simulink model "o_heli3d"  (Simulink 7.7)
settings: Solver=ode1  StartTime=0.0  StopTime=inf  FixedStep=0.002  RelTol=1e-3
values from neighbouring files (symbols this model uses):
  A_kal = Kest.a    [setup_lab_heli_3d_various_controler_with_Kalman_Filter.m]
  B_kal = Kest.b    [setup_lab_heli_3d_various_controler_with_Kalman_Filter.m]
  C = [1,0,0,0,0,0 ... (first row only)    [lab_init.m]    (also in o_lqi.m = [1,0,0,0,0; 0,0,0,0,1])
  C_kal = eye(6)    [setup_lab_heli_3d_various_controler_with_Kalman_Filter.m]
  CMD_ELEV_POS_LIMIT_LOWER = elev_0*180/pi    (= -27.5)    [setup_lab_heli_3d.m]    (also in setup_lab_heli_3d_simple.m; setup_lab_heli_3d_various_controler.m; setup_lab_heli_3d_various_controler_with_Kalman_Filter.m)
  CMD_ELEV_POS_LIMIT_UPPER = -CMD_ELEV_POS_LIMIT_LOWER    (= 27.5)    [setup_lab_heli_3d.m]    (also in setup_lab_heli_3d_simple.m; setup_lab_heli_3d_various_controler.m; setup_lab_heli_3d_various_controler_with_Kalman_Filter.m)
  CMD_RATE_LIMIT = 45.0 * pi / 180    (= 0.785398163397)    [setup_lab_heli_3d.m]    (also in setup_lab_heli_3d_simple.m; setup_lab_heli_3d_various_controler.m; setup_lab_heli_3d_various_controler_with_Kalman_Filter.m)
  D_kal = zeros(6,5)    [setup_lab_heli_3d_various_controler_with_Kalman_Filter.m]
  elev_0 = -27.5*pi/180    (= -0.479965544298)    [setup_lab_heli_3d.m]    (also in setup_lab_heli_3d_simple.m; setup_lab_heli_3d_various_controler.m; setup_lab_heli_3d_various_controler_with_Kalman_Filter.m)
  g = 9.81    [linnlsys.m]
  K_AMP = 3    [setup_lab_heli_3d.m]    (also in setup_lab_heli_3d_simple.m; setup_lab_heli_3d_various_controler.m; setup_lab_heli_3d_various_controler_with_Kalman_Filter.m)
  K_JOYSTICK_X = 40.0    (= 40)    [setup_lab_heli_3d.m]    (also in setup_lab_heli_3d_simple.m; setup_lab_heli_3d_various_controler.m; setup_lab_heli_3d_various_controler_with_Kalman_Filter.m)
  K_JOYSTICK_Y = 45.0    (= 45)    [setup_lab_heli_3d.m]    (also in setup_lab_heli_3d_simple.m; setup_lab_heli_3d_various_controler.m; setup_lab_heli_3d_various_controler_with_Kalman_Filter.m)
  Kr = [L(:,1),L(:,5)]    [o_lqi.m]    (also in setup_lab_heli_3d_various_controler.m = [L eye(2,2)]*A_tot_inv*[zeros(6,3);eye(3,3)]; setup_lab_heli_3d_various_controler_with_Kalman_Filter.m = -V_svd*inv(S_svd)*U_svd')
  L = lqr( Ae, Be, Q, R )    [o_lqi.m]    (also in setup_lab_heli_3d_various_controler.m = Le(:,1:6); setup_lab_heli_3d_various_controler_with_Kalman_Filter.m = lqr( A, B, Q, R ))
  La = 26.0 * 0.0254    (= 0.6604)    [linnlsys.m]
  V = eye(3)    [setup_lab_heli_3d_various_controler_with_Kalman_Filter.m]
  VMAX_AMP = 24    [setup_lab_heli_3d.m]    (also in setup_lab_heli_3d_simple.m; setup_lab_heli_3d_various_controler.m; setup_lab_heli_3d_various_controler_with_Kalman_Filter.m)
  VMAX_DAC = 10    [setup_lab_heli_3d.m]    (also in setup_lab_heli_3d_simple.m; setup_lab_heli_3d_various_controler.m; setup_lab_heli_3d_various_controler_with_Kalman_Filter.m)
  W = diag([1e3 1e3 1e3 1e-3 1e-3 1e-3])    [setup_lab_heli_3d_various_controler_with_Kalman_Filter.m]
  wcf = 2 * pi * 2.5    (= 15.7079632679)    [setup_ads_configuration.m]    (also in setup_lab_heli_3d.m = 125.663706144; setup_lab_heli_3d_simple.m = 125.663706144; setup_lab_heli_3d_various_controler.m = 125.663706144; setup_lab_heli_3d_various_controler_with_Kalman_Filter.m = 125.663706144)
  zetaf = 0.9    [setup_lab_heli_3d.m]    (also in setup_lab_heli_3d_simple.m; setup_lab_heli_3d_various_controler.m; setup_lab_heli_3d_various_controler_with_Kalman_Filter.m)
undefined symbols (not defined in the file or in its folder): ax, ay, az, CMD_TRAVEL_POS_LIMIT_LOWER, CMD_TRAVEL_POS_LIMIT_UPPER, HIL, K_EC_E, K_EC_P, K_EC_T, Kf, Lw, m_b, m_f, m_w, P, p, qc_get_step_size
libraries: quarc_library x5, simulink_extras x4, simulink x3
settings Model: Creator=MLevis  LastModifiedBy=helicopter  SimulationMode=external  ExtModeTrigDuration=10000
settings SolverCC: PositivePriorityOrder=on
settings OptimizationCC: InitFltsAndDblsToZero=on
settings DebuggingCC: SaveWithParameterizedLinksMsg=none  StrictBusMsg=Warning
settings RTWCC: SystemTargetFile=quarc_win64.tlc  TemplateMakefile=quarc_default_tmf  Description=QUARC Win64 Target  ProcessScript=quarc_win64_make_rtw_hook
settings STFCustomTargetCC: TargetPreCompLibLocation=C:\PROGRA~3\QUARC\lib\2011a\win64\release  FunctionExecutionProfile=off  GeneratePreprocessorConditionals=Disable all  SystemTargetFile=quarc_win64.tlc
settings GRTTargetCC: TargetPreCompLibLocation=C:\PROGRA~3\QUARC\lib\2011a\win64\release  ParMdlRefBuildCompliant=off  CompOptLevelCompliant=off  MatFileLogging=off  ExtMode=on  ExtModeMexFile=quarc_comm

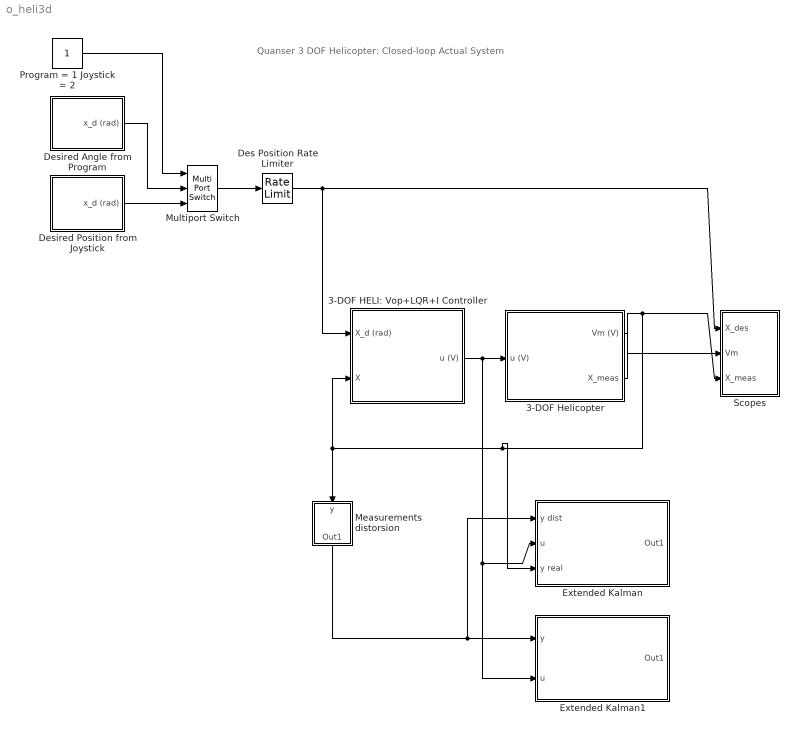
== system o_heli3d ==
  note: Quanser 3 DOF Helicopter:
      | Closed-loop Actual System
  3-DOF HELI: Vop+LQR+I Controller : Subsystem
  3-DOF Helicopter : Subsystem
  Des Position Rate Limiter : RateLimiter  RisingSlewLimit=CMD_RATE_LIMIT  FallingSlewLimit=-CMD_RATE_LIMIT  SampleTimeMode=inherited
  Desired Angle from Program : Subsystem
  Desired Position from Joystick : Subsystem
  Extended Kalman : Subsystem
  Extended Kalman1 : Subsystem
  Measurements distorsion : Subsystem
  Multiport Switch : MultiPortSwitch  Inputs=2  zeroidx=off
  Program = 1 Joystick = 2 : Constant
  Scopes : Subsystem
  wires:
  3-DOF Helicopter/1(Vm (V)) -> Scopes/2(Vm)
  3-DOF Helicopter/2(X_meas) -> Scopes/3(X_meas), 3-DOF HELI: Vop+LQR+I Controller/2(X), Measurements distorsion/1(y), Extended Kalman/3(y real)
  Des Position Rate Limiter/1 -> Scopes/1(X_des), 3-DOF HELI: Vop+LQR+I Controller/1(X_d (rad))
  Program = 1 Joystick = 2/1 -> Multiport Switch/1
  Desired Angle from Program/1(x_d (rad)) -> Multiport Switch/2
  Desired Position from Joystick/1(x_d (rad)) -> Multiport Switch/3
  Multiport Switch/1 -> Des Position Rate Limiter/1
  3-DOF HELI: Vop+LQR+I Controller/1(u (V)) -> 3-DOF Helicopter/1(u (V)), Extended Kalman1/2(u), Extended Kalman/2(u)
  Measurements distorsion/1(Out1) -> Extended Kalman1/1(y), Extended Kalman/1(y dist)

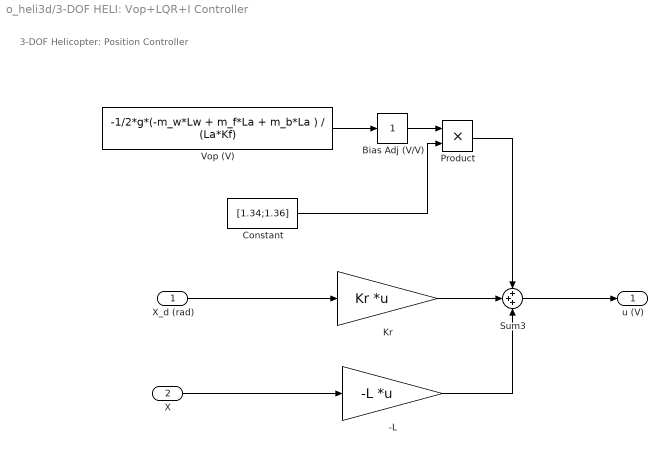
== system o_heli3d/3-DOF HELI: Vop+LQR+I Controller ==
  note: 3-DOF Helicopter: Position Controller
  X_d (rad) : Inport
  X : Inport  Port=2
  -L : Gain  Gain=-L  Multiplication=Matrix(K*u)
  Bias Adj (V/V) : simulink/Math Operations/Slider Gain  SystemSampleTime=-1  low=0  gain=1  high=1
  Constant : Constant  Value=[1.34;1.36]
  Kr : Gain  Gain=Kr  Multiplication=Matrix(K*u)
  Product : Product  RndMeth=Zero
  Sum3 : Sum  Inputs=+++
  Vop (V) : Constant  Value=-1/2*g*(-m_w*Lw + m_f*La + m_b*La ) / (La*Kf)
  u (V) : Outport
  wires:
  X_d (rad)/1 -> Kr/1
  X/1 -> -L/1
  Sum3/1 -> u (V)/1
  Vop (V)/1 -> Bias Adj (V/V)/1
  Bias Adj (V/V)/1 -> Product/1
  Constant/1 -> Product/2
  Product/1 -> Sum3/1
  Kr/1 -> Sum3/2
  -L/1 -> Sum3/3

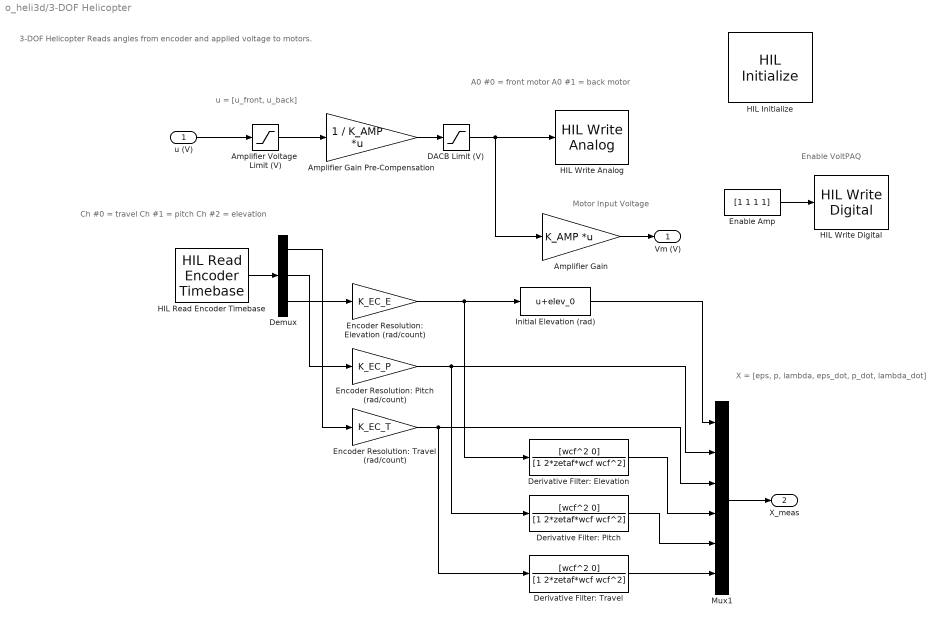
== system o_heli3d/3-DOF Helicopter ==
  note: A0 #0 = front motor
      | A0 #1 = back motor
  note: u = [u_front, u_back]
  note: Motor Input Voltage
  note: 3-DOF Helicopter
      | Reads angles from encoder and applied voltage to motors.
  note: Ch #0 = travel
      | Ch #1 = pitch
      | Ch #2 = elevation
  note: X = [eps, p, lambda, eps_dot, p_dot, lambda_dot]
  note: Enable VoltPAQ
  u (V) : Inport
  Amplifier Gain : Gain  Gain=K_AMP  Multiplication=Matrix(K*u)  SaturateOnIntegerOverflow=on  OutDataTypeStr=Inherit: Same as input  ParamDataTypeStr=Inherit: Same as input
  Amplifier Gain Pre-Compensation : Gain  Gain=1 / K_AMP  Multiplication=Matrix(K*u)  SaturateOnIntegerOverflow=on  OutDataTypeStr=Inherit: Same as input  ParamDataTypeStr=Inherit: Same as input
  Amplifier Voltage  Limit (V) : Saturate  UpperLimit=VMAX_AMP  LowerLimit=-VMAX_AMP
  DACB Limit (V) : Saturate  UpperLimit=VMAX_DAC  LowerLimit=-VMAX_DAC
  Demux : Demux  Outputs=3
  Derivative Filter: Elevation : TransferFcn  Numerator=[wcf^2 0]  Denominator=[1 2*zetaf*wcf wcf^2]
  Derivative Filter: Pitch : TransferFcn  Numerator=[wcf^2 0]  Denominator=[1 2*zetaf*wcf wcf^2]
  Derivative Filter: Travel : TransferFcn  Numerator=[wcf^2 0]  Denominator=[1 2*zetaf*wcf wcf^2]
  Enable Amp : Constant  Value=[1 1 1 1]
  Encoder Resolution: Elevation (rad/count) : Gain  Gain=K_EC_E
  Encoder Resolution: Pitch (rad/count) : Gain  Gain=K_EC_P
  Encoder Resolution: Travel (rad/count) : Gain  Gain=K_EC_T
  HIL Initialize : quarc_library/Data Acquisition/Generic/Configuration/HIL Initialize  object_name=HIL-1  board_type=q8_usb  board_number=0  board_options=update_rate=normal  exclusive=off  active=on  hardware_clocks=[0:2]  clock_modes=[]  initial_clock_frequencies=[]  set_clock_params_at_start=off  set_clock_params_at_switch_in=off  set_clock_frequencies_at_start=off  set_clock_frequencies_at_switch_in=off  analog_input_channels=[0:7]  analog_input_maximums=10  analog_input_minimums=-10  set_analog_input_params_at_start=on  set_analog_input_params_at_switch_in=off  analog_output_channels=[0:7]  analog_output_maximums=10  analog_output_minimums=-10  initial_analog_outputs=[0]  final_analog_outputs=[0]  watchdog_analog_outputs=0  set_analog_output_params_at_start=on  set_analog_output_params_at_switch_in=off  set_analog_outputs_at_start=on  set_analog_outputs_at_switch_in=off  set_analog_outputs_at_terminate=on  set_analog_outputs_at_switch_out=off  set_analog_outputs_on_watchdog=off  digital_input_channels=[4:7]  digital_output_channels=[0:3]  digital_output_configuration=[]  initial_digital_outputs=[0]  final_digital_outputs=[0]  watchdog_digital_outputs=[0]  set_digital_output_params_at_start=off  set_digital_output_params_at_switch_in=off  set_digital_outputs_at_start=on  set_digital_outputs_at_switch_in=off  set_digital_outputs_at_terminate=on  set_digital_outputs_at_switch_out=off  set_digital_outputs_on_watchdog=off  encoder_channels=[0:7]  quadrature=[4]  encoder_filter_frequency=[]  initial_encoder_counts=[0]  set_encoder_params_at_start=on  set_encoder_params_at_switch_in=off  set_encoder_counts_at_start=on  set_encoder_counts_at_switch_in=off  pwm_channels=[0:7]  pwm_modes=0  pwm_frequency=99.532799999999995e6/4095  pwm_configuration=[0]  pwm_alignment=[0]  pwm_polarity=[1]  pwm_leading_deadband=[0]  pwm_trailing_deadband=[0]  initial_pwm_outputs=[0]  final_pwm_outputs=[0]  watchdog_pwm_outputs=[0]  set_pwm_params_at_start=on  set_pwm_params_at_switch_in=off  set_pwm_outputs_at_start=on  set_pwm_outputs_at_switch_in=off  set_pwm_outputs_at_terminate=on  set_pwm_outputs_at_switch_out=off  set_pwm_outputs_on_watchdog=off  other_output_channels=[]  initial_other_outputs=[]  final_other_outputs=[]  watchdog_other_outputs=[]  set_other_outputs_at_start=off  set_other_outputs_at_switch_in=off  set_other_outputs_at_terminate=off  set_other_outputs_at_switch_out=off  set_other_outputs_on_watchdog=off
  HIL Read Encoder Timebase : quarc_library/Data Acquisition/Generic/Timebases/HIL Read Encoder Timebase  object_name=HIL-1  clock=0  channels=[0:2]  samples_in_buffer=max(ceil(1/qc_get_step_size), 1)  active=on  vector_output=on  data_type_mode=Inherit via back propagation  data_type=double
  HIL Write Analog : quarc_library/Data Acquisition/Generic/Immediate I//O/HIL Write Analog  object_name=HIL-1  channels=[0,1]  sample_time=-1  active=off  vector_input=on
  HIL Write Digital : quarc_library/Data Acquisition/Generic/Immediate I//O/HIL Write Digital  object_name=HIL-1  channels=[0:3]  sample_time=-1  active=off  vector_input=on
  Initial Elevation (rad) : Bias  Bias=elev_0
  Mux1 : Mux  Inputs=6
  Vm (V) : Outport
  X_meas : Outport  Port=2
  wires:
  HIL Read Encoder Timebase/1 -> Demux/1
  Mux1/1 -> X_meas/1
  Amplifier Gain Pre-Compensation/1 -> DACB Limit (V)/1
  Amplifier Voltage  Limit (V)/1 -> Amplifier Gain Pre-Compensation/1
  Amplifier Gain/1 -> Vm (V)/1
  u (V)/1 -> Amplifier Voltage  Limit (V)/1
  DACB Limit (V)/1 -> Amplifier Gain/1, HIL Write Analog/1
  Demux/3 -> Encoder Resolution: Elevation (rad/count)/1
  Demux/1 -> Encoder Resolution: Travel (rad/count)/1
  Demux/2 -> Encoder Resolution: Pitch (rad/count)/1
  Encoder Resolution: Elevation (rad/count)/1 -> Derivative Filter: Elevation/1, Initial Elevation (rad)/1
  Encoder Resolution: Pitch (rad/count)/1 -> Mux1/2, Derivative Filter: Pitch/1
  Encoder Resolution: Travel (rad/count)/1 -> Mux1/3, Derivative Filter: Travel/1
  Derivative Filter: Elevation/1 -> Mux1/4
  Derivative Filter: Pitch/1 -> Mux1/5
  Derivative Filter: Travel/1 -> Mux1/6
  Initial Elevation (rad)/1 -> Mux1/1
  Enable Amp/1 -> HIL Write Digital/1

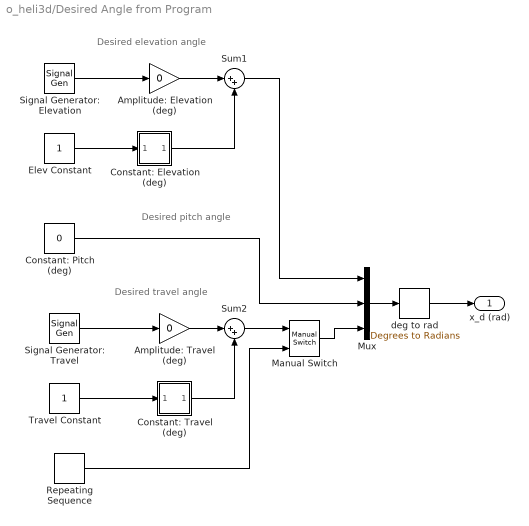
== system o_heli3d/Desired Angle from Program ==
  note: Desired travel angle
  note: Desired elevation angle
  note: Desired pitch angle
  Amplitude: Elevation (deg) : Gain  Gain=0
  Amplitude: Travel (deg) : Gain  Gain=0
  Constant: Elevation (deg) : Subsystem  LoadFcn=slideg Load  StartFcn=slideg StartFcn  StopFcn=slideg StopFcn  mask(Slider Gain){low=-27.5, gain=0, high=100}
      settings: CopyFcn=slideg Copy  DeleteFcn=slideg DeleteBlock  NameChangeFcn=slideg NameChange  OpenFcn=slideg Open  CloseFcn=slideg Close  ParentCloseFcn=slideg ParentClose
      mask Display: disp(gain)
  Constant: Pitch (deg) : Constant  Value=0
  Constant: Travel (deg) : Subsystem  LoadFcn=slideg Load  StartFcn=slideg StartFcn  StopFcn=slideg StopFcn  mask(Slider Gain){low=-90, gain=0, high=90}
      settings: CopyFcn=slideg Copy  DeleteFcn=slideg DeleteBlock  NameChangeFcn=slideg NameChange  OpenFcn=slideg Open  CloseFcn=slideg Close  ParentCloseFcn=slideg ParentClose
      mask Display: disp(gain)
  Elev Constant : Constant
  Manual Switch : simulink/Signal Routing/Manual Switch  SystemSampleTime=-1  sw=1  action=0  varsize=off
  Mux : Mux  Inputs=3
  Repeating Sequence : simulink/Sources/Repeating Sequence  SystemSampleTime=-1  rep_seq_t="[0  15 16  30  45  46 60 ]"  rep_seq_y="[0 0 30 30  30 0 0 ]"
  Signal Generator: Elevation : SignalGenerator  WaveForm=square  Frequency=0.04
  Signal Generator: Travel : SignalGenerator  WaveForm=square  Frequency=0.03
  Sum1 : Sum  Inputs=|++
  Sum2 : Sum  Inputs=|++
  Travel Constant : Constant
  deg to rad : simulink_extras/Transformations/Degrees to Radians  SystemSampleTime=-1
  x_d (rad) : Outport
  wires:
  deg to rad/1 -> x_d (rad)/1
  Signal Generator: Travel/1 -> Amplitude: Travel (deg)/1
  Amplitude: Travel (deg)/1 -> Sum2/1
  Travel Constant/1 -> Constant: Travel (deg)/1(In1)
  Sum1/1 -> Mux/1
  Signal Generator: Elevation/1 -> Amplitude: Elevation (deg)/1
  Amplitude: Elevation (deg)/1 -> Sum1/1
  Mux/1 -> deg to rad/1
  Constant: Pitch (deg)/1 -> Mux/2
  Elev Constant/1 -> Constant: Elevation (deg)/1(In1)
  Constant: Elevation (deg)/1(Out1) -> Sum1/2
  Constant: Travel (deg)/1(Out1) -> Sum2/2
  Sum2/1 -> Manual Switch/1
  Manual Switch/1 -> Mux/3
  Repeating Sequence/1 -> Manual Switch/2

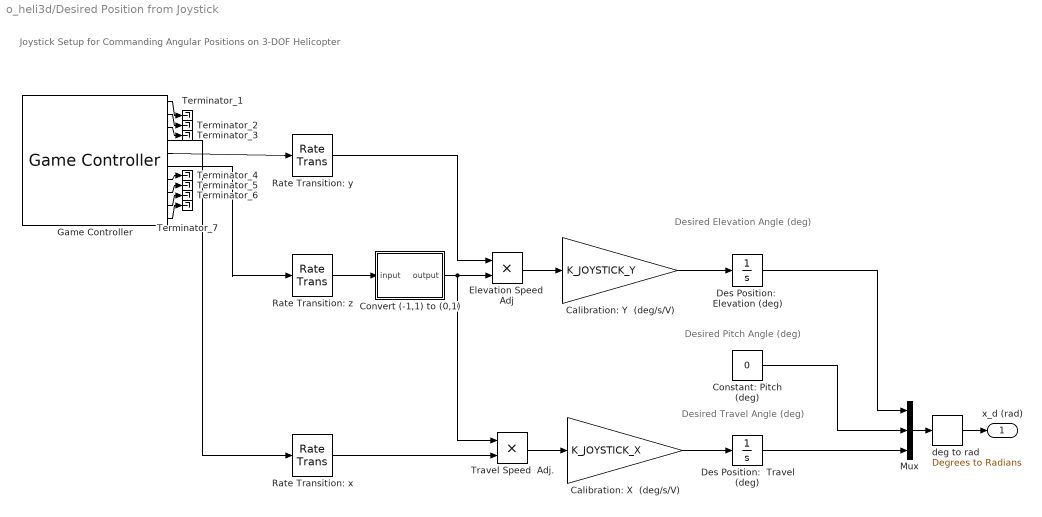
== system o_heli3d/Desired Position from Joystick ==
  note: Desired Pitch Angle (deg)
  note: Desired Elevation Angle (deg)
  note: Desired Travel Angle (deg)
  note: Joystick Setup for Commanding Angular Positions on 3-DOF Helicopter
  Calibration: X  (deg/s/V) : Gain  Gain=K_JOYSTICK_X
  Calibration: Y  (deg/s/V) : Gain  Gain=K_JOYSTICK_Y
  Constant: Pitch (deg) : Constant  Value=0
  Convert (-1,1) to (0,1) : Subsystem
  Des Position:  Elevation (deg) : Integrator  InitialCondition=elev_0*180/pi  LimitOutput=on  UpperSaturationLimit=CMD_ELEV_POS_LIMIT_UPPER  LowerSaturationLimit=CMD_ELEV_POS_LIMIT_LOWER
  Des Position:  Travel (deg) : Integrator  UpperSaturationLimit=CMD_TRAVEL_POS_LIMIT_UPPER  LowerSaturationLimit=CMD_TRAVEL_POS_LIMIT_LOWER
  Elevation Speed  Adj : Product  RndMeth=Zero
  Game Controller : quarc_library/Devices/Peripherals/Target/Game Controller  controller=1  buffer_size=12  deadzone=[]  saturation=[]  sample_time=max(qc_get_step_size, 0.01)  auto_center=off  enabled=on
  Mux : Mux  Inputs=3
  Rate Transition: x : RateTransition
  Rate Transition: y : RateTransition
  Rate Transition: z : RateTransition
  Terminator_{1..7} (7 alike) : Terminator
  Travel Speed  Adj. : Product  RndMeth=Zero
  deg to rad : simulink_extras/Transformations/Degrees to Radians  SystemSampleTime=-1
  x_d (rad) : Outport
  wires:
  Des Position:  Elevation (deg)/1 -> Mux/1
  Constant: Pitch (deg)/1 -> Mux/2
  Des Position:  Travel (deg)/1 -> Mux/3
  Mux/1 -> deg to rad/1
  deg to rad/1 -> x_d (rad)/1
  Calibration: X  (deg/s/V)/1 -> Des Position:  Travel (deg)/1
  Travel Speed  Adj./1 -> Calibration: X  (deg/s/V)/1
  Elevation Speed  Adj/1 -> Calibration: Y  (deg/s/V)/1
  Calibration: Y  (deg/s/V)/1 -> Des Position:  Elevation (deg)/1
  Convert (-1,1) to (0,1)/1(output) -> Travel Speed  Adj./1, Elevation Speed  Adj/2
  Rate Transition: z/1 -> Convert (-1,1) to (0,1)/1(input)
  Rate Transition: y/1 -> Elevation Speed  Adj/1
  Rate Transition: x/1 -> Travel Speed  Adj./2
  Game Controller/5 -> Rate Transition: y/1
  Game Controller/6 -> Rate Transition: z/1
  Game Controller/4 -> Rate Transition: x/1
  Game Controller/1 -> Terminator_1/1
  Game Controller/2 -> Terminator_2/1
  Game Controller/3 -> Terminator_3/1
  Game Controller/7 -> Terminator_4/1
  Game Controller/8 -> Terminator_5/1
  Game Controller/9 -> Terminator_6/1
  Game Controller/10 -> Terminator_7/1

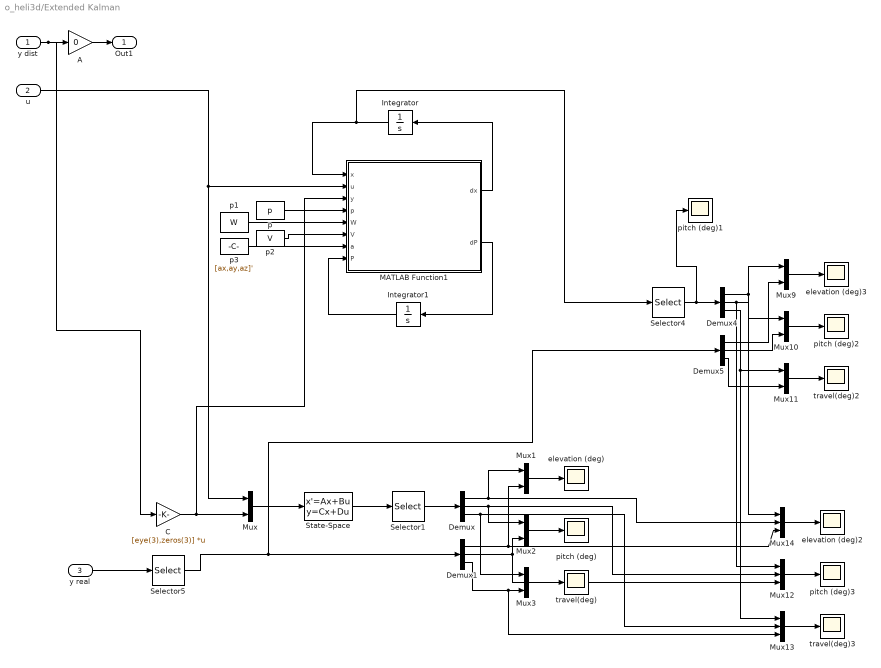
== system o_heli3d/Extended Kalman ==
  y dist : Inport
  u : Inport  Port=2
  y real : Inport  Port=3
  A : Gain  Gain=0
  C : Gain  Gain=[eye(3),zeros(3)]  Multiplication=Matrix(K*u)
  Demux{,1,4..5} (4 alike) : Demux  Outputs=3
  Integrator : Integrator
  Integrator1 : Integrator  InitialCondition=P
  MATLAB Function1 : Stateflow chart  TreatAsAtomicUnit=on
  Mux{,1..3,9..11} (7 alike) : Mux  Inputs=2
  Mux12 : Mux  Inputs=3
  Mux13 : Mux  Inputs=3
  Mux14 : Mux  Inputs=3
  Selector1 : Selector  InputPortWidth=6  IndexOptions=Index vector (dialog)  Indices=[1 2 3]  OutputSizes=1
  Selector4 : Selector  InputPortWidth=6  IndexOptions=Index vector (dialog)  Indices=[1 2 3]  OutputSizes=1
  Selector5 : Selector  InputPortWidth=6  IndexOptions=Index vector (dialog)  Indices=[1,2,3]  OutputSizes=1
  State-Space : StateSpace  A=A_kal  B=B_kal  C=C_kal  D=D_kal
  elevation (deg) : Scope
      settings: TickLabels=on  TimeRange=140  YMin=-1  YMax=17  SaveName=ScopeData7  DataFormat=Array
  elevation (deg)2 : Scope
      settings: TickLabels=on  TimeRange=140  YMin=-0.08475  YMax=-0.081  SaveName=ScopeData3  DataFormat=Array
  elevation (deg)3 : Scope
      settings: TickLabels=on  TimeRange=140  YMin=-0.21775  YMax=-0.2145  SaveName=ScopeData5  DataFormat=Array
  p : Constant  Value=p
  p1 : Constant  Value=W
  p2 : Constant  Value=V
  p3 : Constant  Value=[ax,ay,az]'
  pitch (deg){,1..3} (4 alike) : Scope
      pitch (deg) settings: TickLabels=on  TimeRange=20  YMin=0.6595  YMax=0.66015  SaveName=ScopeData8  DataFormat=Array
      pitch (deg)1 settings: TickLabels=on  TimeRange=20  YMin=0.0306  YMax=0.0323  SaveName=ScopeData17  DataFormat=Array
      pitch (deg)2 settings: TickLabels=on  TimeRange=20  YMin=0.006  YMax=0.03  SaveName=ScopeData6  DataFormat=Array
      pitch (deg)3 settings: TickLabels=on  TimeRange=20  YMin=-0.0025  YMax=0.04  SaveName=ScopeData14  DataFormat=Array
  travel(deg) : Scope
      settings: TickLabels=on  TimeRange=20  YMin=0  YMax=14  SaveName=ScopeData9  DataFormat=Array
  travel(deg)2 : Scope
      settings: TickLabels=on  TimeRange=20  YMin=0.339547  YMax=0.375289  SaveName=ScopeData13  DataFormat=Array
  travel(deg)3 : Scope
      settings: TickLabels=on  TimeRange=20  YMin=-27.5  YMax=2.5  SaveName=ScopeData15  DataFormat=Array
  Out1 : Outport
  wires:
  y dist/1 -> A/1, C/1
  A/1 -> Out1/1
  u/1 -> Mux/1, MATLAB Function1/2(u)
  State-Space/1 -> Selector1/1
  C/1 -> Mux/2, MATLAB Function1/3(y)
  Mux/1 -> State-Space/1
  Selector1/1 -> Demux/1
  Mux1/1 -> elevation (deg)/1
  Mux2/1 -> pitch (deg)/1
  Mux3/1 -> travel(deg)/1
  Demux/1 -> Mux1/1, Mux14/2
  Demux/2 -> Mux2/1, Mux12/2
  Demux/3 -> Mux3/1, Mux13/2
  Demux1/1 -> Mux1/2, Mux14/3
  Demux1/2 -> Mux2/2, Mux12/3
  Demux1/3 -> Mux3/2, Mux13/3
  Mux9/1 -> elevation (deg)3/1
  Mux10/1 -> pitch (deg)2/1
  Mux11/1 -> travel(deg)2/1
  Demux4/1 -> Mux9/1, Mux14/1
  Demux4/2 -> Mux10/1, Mux12/1
  Demux4/3 -> Mux11/1, Mux13/1
  Demux5/1 -> Mux9/2
  Demux5/2 -> Mux10/2
  Demux5/3 -> Mux11/2
  Selector4/1 -> Demux4/1, pitch (deg)1/1
  Mux14/1 -> elevation (deg)2/1
  Mux12/1 -> pitch (deg)3/1
  Mux13/1 -> travel(deg)3/1
  Selector5/1 -> Demux1/1, Demux5/1
  Integrator/1 -> MATLAB Function1/1(x), Selector4/1
  p/1 -> MATLAB Function1/4(p)
  p2/1 -> MATLAB Function1/6(V)
  p1/1 -> MATLAB Function1/5(W)
  p3/1 -> MATLAB Function1/7(a)
  MATLAB Function1/1(dx) -> Integrator/1
  Integrator1/1 -> MATLAB Function1/8(P)
  MATLAB Function1/2(dP) -> Integrator1/1
  y real/1 -> Selector5/1

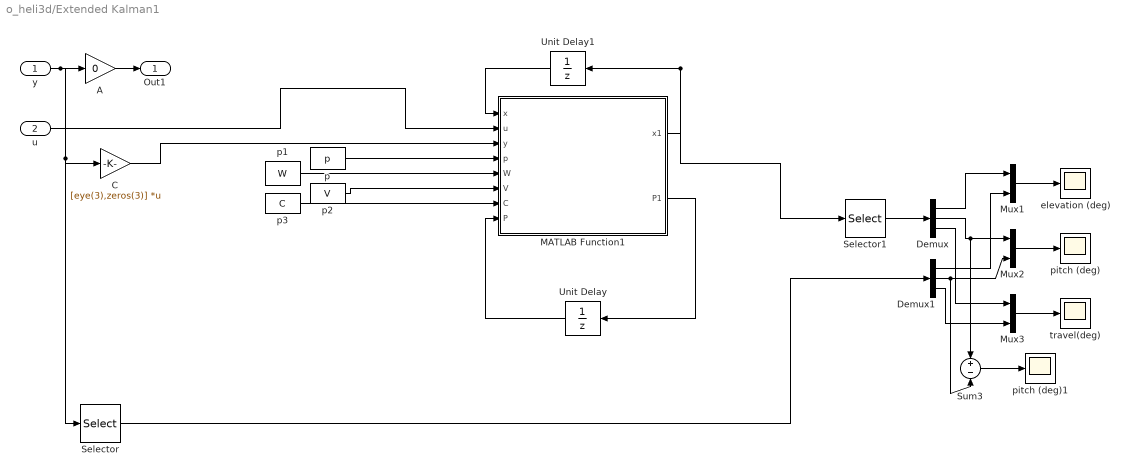
== system o_heli3d/Extended Kalman1 ==
  y : Inport
  u : Inport  Port=2
  A : Gain  Gain=0
  C : Gain  Gain=[eye(3),zeros(3)]  Multiplication=Matrix(K*u)
  Demux : Demux  Outputs=3
  Demux1 : Demux  Outputs=3
  MATLAB Function1 : Stateflow chart  TreatAsAtomicUnit=on
  Mux1 : Mux  Inputs=2
  Mux2 : Mux  Inputs=2
  Mux3 : Mux  Inputs=2
  Selector : Selector  InputPortWidth=6  IndexOptions=Index vector (dialog)  Indices=[1,2,3]  OutputSizes=1
  Selector1 : Selector  InputPortWidth=6  IndexOptions=Index vector (dialog)  Indices=[1 2 3]  OutputSizes=1
  Sum3 : Sum  Inputs=+|-
  Unit Delay : UnitDelay  X0=P  SampleTime=-1
  Unit Delay1 : UnitDelay  SampleTime=-1
  elevation (deg) : Scope
      settings: TickLabels=on  TimeRange=140  YMin=-0.25  YMax=0.5  SaveName=ScopeData10  DataFormat=Array
  p : Constant  Value=p
  p1 : Constant  Value=W
  p2 : Constant  Value=V
  p3 : Constant  Value=C
  pitch (deg) : Scope
      settings: TickLabels=on  TimeRange=20  YMin=-0.0025  YMax=0.04  SaveName=ScopeData11  DataFormat=Array
  pitch (deg)1 : Scope
      settings: TickLabels=on  TimeRange=20  YMin=-0.14  YMax=-0.01  SaveName=ScopeData16  DataFormat=Array
  travel(deg) : Scope
      settings: TickLabels=on  TimeRange=20  YMin=-0.55  YMax=0.1  SaveName=ScopeData12  DataFormat=Array
  Out1 : Outport
  wires:
  Selector/1 -> Demux1/1
  A/1 -> Out1/1
  y/1 -> A/1, Selector/1, C/1
  MATLAB Function1/1(x1) -> Unit Delay1/1, Selector1/1
  Unit Delay1/1 -> MATLAB Function1/1(x)
  MATLAB Function1/2(P1) -> Unit Delay/1
  Unit Delay/1 -> MATLAB Function1/8(P)
  p/1 -> MATLAB Function1/4(p)
  p2/1 -> MATLAB Function1/6(V)
  p1/1 -> MATLAB Function1/5(W)
  p3/1 -> MATLAB Function1/7(C)
  Selector1/1 -> Demux/1
  Mux1/1 -> elevation (deg)/1
  Mux2/1 -> pitch (deg)/1
  Mux3/1 -> travel(deg)/1
  Demux/1 -> Mux1/1
  Demux/2 -> Mux2/1, Sum3/1
  Demux/3 -> Mux3/1
  Demux1/1 -> Mux1/2
  Demux1/2 -> Mux2/2, Sum3/2
  Demux1/3 -> Mux3/2
  C/1 -> MATLAB Function1/3(y)
  Sum3/1 -> pitch (deg)1/1
  u/1 -> MATLAB Function1/2(u)

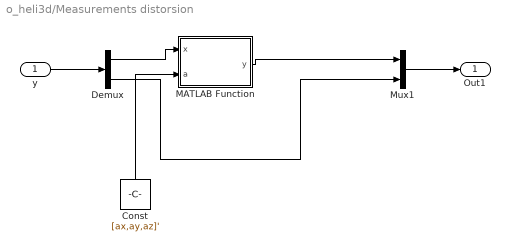
== system o_heli3d/Measurements distorsion ==
  y : Inport
  Const : Constant  Value=[ax,ay,az]'
  Demux : Demux  Outputs=2
  MATLAB Function : Stateflow chart  TreatAsAtomicUnit=on
  Mux1 : Mux  Inputs=2
  Out1 : Outport
  wires:
  y/1 -> Demux/1
  Demux/1 -> MATLAB Function/1(x)
  Demux/2 -> Mux1/2
  Mux1/1 -> Out1/1
  MATLAB Function/1(y) -> Mux1/1
  Const/1 -> MATLAB Function/2(a)

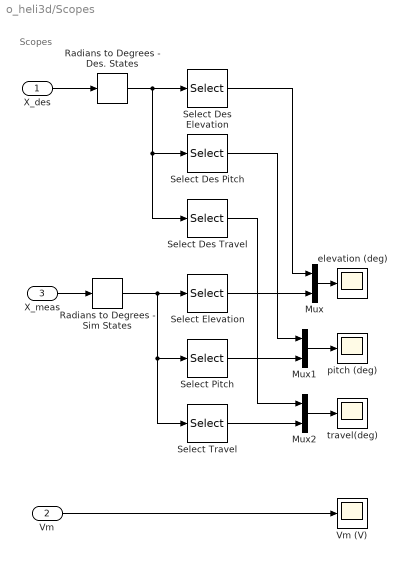
== system o_heli3d/Scopes ==
  note: Scopes
  X_des : Inport
  Vm : Inport  Port=2
  X_meas : Inport  Port=3
  Mux : Mux  Inputs=2
  Mux1 : Mux  Inputs=2
  Mux2 : Mux  Inputs=2
  Radians to Degrees - Des. States : simulink_extras/Transformations/Radians to Degrees  SystemSampleTime=-1
  Radians to Degrees - Sim States : simulink_extras/Transformations/Radians to Degrees  SystemSampleTime=-1
  Select Des Elevation : Selector  InputPortWidth=3  IndexOptions=Index vector (dialog)  Indices=1  OutputSizes=1
  Select Des Pitch : Selector  InputPortWidth=3  IndexOptions=Index vector (dialog)  Indices=2  OutputSizes=1
  Select Des Travel : Selector  InputPortWidth=3  IndexOptions=Index vector (dialog)  Indices=3  OutputSizes=1
  Select Elevation : Selector  InputPortWidth=6  IndexOptions=Index vector (dialog)  Indices=1  OutputSizes=1
  Select Pitch : Selector  InputPortWidth=6  IndexOptions=Index vector (dialog)  Indices=2  OutputSizes=1
  Select Travel : Selector  InputPortWidth=6  IndexOptions=Index vector (dialog)  Indices=3  OutputSizes=1
  Vm (V) : Scope
      settings: TickLabels=on  TimeRange=20  YMin=3  YMax=20  SaveName=ScopeData4  DataFormat=Array
  elevation (deg) : Scope
      settings: TickLabels=on  TimeRange=140  YMin=-15  DataFormat=Array
  pitch (deg) : Scope
      settings: TickLabels=on  TimeRange=20  YMin=-35  YMax=40  DataFormat=Array
  travel(deg) : Scope
      settings: TickLabels=on  TimeRange=20  YMin=-20  YMax=2.5  SaveName=ScopeData2  DataFormat=Array
  wires:
  Select Des Travel/1 -> Mux2/1
  Select Des Pitch/1 -> Mux1/1
  Select Des Elevation/1 -> Mux/1
  Radians to Degrees - Des. States/1 -> Select Des Travel/1, Select Des Pitch/1, Select Des Elevation/1
  Select Travel/1 -> Mux2/2
  Select Pitch/1 -> Mux1/2
  Select Elevation/1 -> Mux/2
  Mux2/1 -> travel(deg)/1
  Radians to Degrees - Sim States/1 -> Select Travel/1, Select Pitch/1, Select Elevation/1
  Vm/1 -> Vm (V)/1
  Mux1/1 -> pitch (deg)/1
  Mux/1 -> elevation (deg)/1
  X_meas/1 -> Radians to Degrees - Sim States/1
  X_des/1 -> Radians to Degrees - Des. States/1

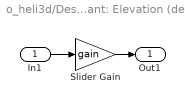
== system o_heli3d/Desired Angle from Program/Constant: Elevation (deg) ==
  In1 : Inport
  Slider Gain : Gain  Gain=gain  SaturateOnIntegerOverflow=on  OutDataTypeStr=Inherit: Same as input  ParamDataTypeStr=Inherit: Same as input
  Out1 : Outport
  wires:
  In1/1 -> Slider Gain/1
  Slider Gain/1 -> Out1/1

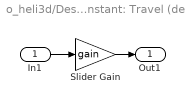
== system o_heli3d/Desired Angle from Program/Constant: Travel (deg) ==
  In1 : Inport
  Slider Gain : Gain  Gain=gain  SaturateOnIntegerOverflow=on  OutDataTypeStr=Inherit: Same as input  ParamDataTypeStr=Inherit: Same as input
  Out1 : Outport
  wires:
  In1/1 -> Slider Gain/1
  Slider Gain/1 -> Out1/1

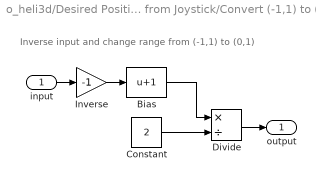
== system o_heli3d/Desired Position from Joystick/Convert (-1,1) to (0,1) ==
  note: Inverse input and change range from (-1,1) to (0,1)
  input : Inport
  Bias : Bias  Bias=1
  Constant : Constant  Value=2
  Divide : Product  Inputs=*/
  Inverse : Gain  Gain=-1
  output : Outport
  wires:
  Constant/1 -> Divide/2
  Bias/1 -> Divide/1
  input/1 -> Inverse/1
  Divide/1 -> output/1
  Inverse/1 -> Bias/1

== matlab function Measurements distorsion/MATLAB Function ==
  data: x input double; y output double; a input double
function y = fcn(x,a)
%#codegen

u = zeros(3,1);
y = zeros(3,1);

u(1,1) = 0.66*cos(x(3))*cos(x(1));
u(2,1) = 0.66*sin(x(3))*cos(x(1));
u(3,1) = 0.66*sin(x(1));




y(1) = sum(u.^2);
y(2) = 0.66;
y(3) = x(2);

== matlab function Extended Kalman1/MATLAB Function1 ==
  data: x input double; u input double; x1 output double; y input double; p input double; W input double; V input double; C input double; P input double; P1 output double
function [x1,P1] = ekalman(x,u,y,p,W,V,C,P)


x1 = [0,0,0,0,0,0]';
P1 = zeros(6);



%
% Discretize nonlinear coninuous model around working point:
%
% ddx = zeros(6,1);
% ddu = zeros(6,1);
% 
% ddx(1,1) = x(4);
% ddx(2,1) = x(5);
% ddx(3,1) = x(6);
% ddx(4,1) = p(1)*cos(x(1))+p(2)*sin(x(1))+p(3)*x(4);
% ddx(5,1) = p(5)*cos(x(2))+p(6)*sin(x(2))+p(7)*x(5);
% ddx(6,1) = p(9)*x(6);
% 
% 
% ddu(1,1) = 0;
% ddu(2,1) = 0;
% ddu(3,1) = 0;
% ddu(4,1) = u(1)*p(4)*cos(x(2)) +  u(2)*p(4)*cos(x(2));
% ddu(5,1) = p(8)*u(1) - p(8)*u(2);
% ddu(6,1) = u(1)*p(10)*sin(x(2)) +  u(2)*p(10)*sin(x(2));


A_c = [                                                                                        0,                                                                                            0, 0,      1,     0,      0;
                                                                                         0,                                                                                                   0, 0,      0,     1,      0;
                                                                                         0,                                                                                                   0, 0,      0,     0,      1;
  (5108936187301295*sin(x(1)))/281474976710656 - (2161496095226779*cos(x(1)))/1125899906842624, - (6573623267668065*u(1)*sin(x(2)))/72057594037927936 - (6573623267668065*u(2)*sin(x(2)))/72057594037927936, 0, -1/860,     0,      0;
                                                                                         0,                                                                               -(16677*cos(x(2)))/1000, 0,      0, -1/44,      0;
                                                                                         0, - (3447143908655205*u(1)*cos(x(2)))/36028797018963968 - (3447143908655205*u(2)*cos(x(2)))/36028797018963968, 0,      0,     0, -1/164];

B_c = [                                      0,                                             0;
                                              0,                                             0;
                                              0,                                             0;
   (6573623267668065*cos(x(2)))/72057594037927936,  (6573623267668065*cos(x(2)))/72057594037927936;
                                    24003/50000,                                  -24003/50000;
  -(3447143908655205*sin(x(2)))/36028797018963968, -(3447143908655205*sin(x(2)))/36028797018963968];

[~,n] = size(A_c);
[~,nb] = size(B_c);
s = expm([[A_c B_c]*0.002; zeros(nb,n+nb)]);
A_d = s(1:n,1:n);
B_d = s(1:n,n+1:n+nb);


%
% Predict
%

% Prediction
x = A_d*x + B_d*u;
% x = x + 0.002*(ddx+ddu);

% Predicted estimate covariance
P = A_d*P*A_d'+W;


%
% Update
%

% Measurement residual
y = y(:)- C*x(:);

% Residual covariance
S = C*P*C' + V;

% Near-Optimal Kalman gain
K = P*C'*inv(S);
 
% Updated state estimate
x1 = x + K*y;
 
P1 = (eye(length(P))-K*C)*P;

== matlab function Extended Kalman/MATLAB Function1 ==
  data: x input double; u input double; dx output double; y input double; p input double; W input double; V input double; a input double; P input double; dP output double
function [dx,dP] = ekalman(x,u,y,p,W,V,a,P)

dx = zeros(6,1);
dP = zeros(6);

ddx = zeros(6,1);
ddu = zeros(6,1);

ddx(1,1) = x(4);
ddx(2,1) = x(5);
ddx(3,1) = x(6);
ddx(4,1) = p(1)*cos(x(1))+p(2)*sin(x(1))+p(3)*x(4);
ddx(5,1) = p(5)*cos(x(2))+p(6)*sin(x(2))+p(7)*x(5);
ddx(6,1) = p(9)*x(6);


ddu(1,1) = 0;
ddu(2,1) = 0;
ddu(3,1) = 0;
ddu(4,1) = u(1)*p(4)*cos(x(2)) +  u(2)*p(4)*cos(x(2));
ddu(5,1) = p(8)*u(1) - p(8)*u(2);
ddu(6,1) = u(1)*p(10)*sin(x(2)) +  u(2)*p(10)*sin(x(2));



F = [                                                                                        0,                                                                                            0, 0,      1,     0,      0;
                                                                                         0,                                                                                                   0, 0,      0,     1,      0;
                                                                                         0,                                                                                                   0, 0,      0,     0,      1;
  (5108936187301295*sin(x(1)))/281474976710656 - (2161496095226779*cos(x(1)))/1125899906842624, - (6573623267668065*u(1)*sin(x(2)))/72057594037927936 - (6573623267668065*u(2)*sin(x(2)))/72057594037927936, 0, -1/860,     0,      0;
                                                                                         0,                                                                               -(16677*cos(x(2)))/1000, 0,      0, -1/44,      0;
                                                                                         0, - (3447143908655205*u(1)*cos(x(2)))/36028797018963968 - (3447143908655205*u(2)*cos(x(2)))/36028797018963968, 0,      0,     0, -1/164];

                                                                   
H = [ 2*0.66*cos(x(3))*sin(x(1))*(a(1) - 0.66*cos(x(1))*cos(x(3))) - 2*0.66*cos(x(1))*(a(3) - 0.66*sin(x(1))) + 2*0.66*sin(x(1))*sin(x(3))*(a(2) - 0.66*cos(x(1))*sin(x(3))), 0, 2*0.66*cos(x(1))*sin(x(3))*(a(1) - 0.66*cos(x(1))*cos(x(3))) - 2*0.66*cos(x(1))*cos(x(3))*(a(2) - 0.66*cos(x(1))*sin(x(3))), 0, 0, 0;
                                      - 2*cos(x(1))*sin(x(1))*0.66^2*cos(x(3))^2 - 2*cos(x(1))*sin(x(1))*0.66^2*sin(x(3))^2 + 2*cos(x(1))*sin(x(1))*0.66^2, 0,                                                                                                   0, 0, 0, 0;
                                      0,1,0,0,0,0];

K = P*H'/V;

hx = zeros(3,1);

hx(1) = (a(1) - 0.66*cos(x(1))*cos(x(3)))^2 + (a(2) - 0.66*cos(x(1))*sin(x(3)))^2 + (a(3) - 0.66*sin(x(1)))^2; 
hx(2) = 0.66^2*cos(x(1))^2*cos(x(3))^2 + 0.66^2*cos(x(1))^2*sin(x(3))^2 + 0.66^2*sin(x(1))^2
hx(3) = x(2);

dx = ddx + ddu + K*(y(:)-hx(:));

dP = F*P+P*F'-K*H*P+W;
